simulink model "hak"  (R2023b)
settings: Solver=VariableStepAuto  StartTime=0.0  StopTime=10  RelTol=1e-3
libraries: mpclib x1, cstblocks x1
settings Model: Creator=serga  LastModifiedBy=serga

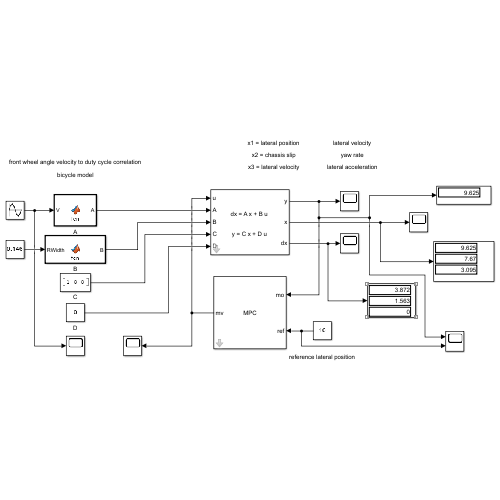
[thumbnail: Simulink's stored preview of the top-level diagram]
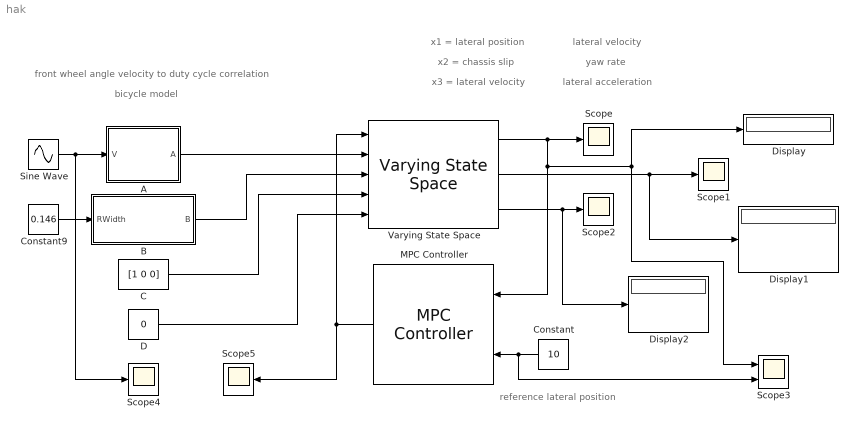
== system hak ==
  note: bicycle model
  note: front wheel angle velocity to duty cycle correlation
  note: reference lateral position
  note: lateral acceleration
  note: yaw rate
  note: lateral velocity
  note: x3 = lateral velocity
  note: x2 = chassis slip
  note: x1 = lateral position
  A : MATLAB Function  TreatAsAtomicUnit=on
  B : MATLAB Function  TreatAsAtomicUnit=on
  C : Constant  Value=[1 0 0]  VectorParams1D=off
  Constant : Constant  Value=10
  Constant9 : Constant  Value=0.146
  D : Constant  Value=0  VectorParams1D=off
  Display : Display
  Display1 : Display
  Display2 : Display
  MPC Controller : mpclib/MPC Controller  SCDEnableBlockLinearizationSpecification=on  mpcobj=mpc1  is_multiple=0  enable_value=0  return_u0=off  updateMPCinCallerWorkspace=on  md_inport=off  mv_inport=off  uref_inport=off  return_cost=off  return_mvseq=off  return_qpstatus=off  return_xseq=off  return_state=off  return_ovseq=off  state_inport=off  umin_inport=off  umax_inport=off  ymin_inport=off  ymax_inport=off  cc_inport=off  ywt_inport=off  uwt_inport=off  duwt_inport=off  rhoeps_inport=off  pm_inport=off  MaximumP=10  HorizonChoice=FixedHorizon  n_ts=0.1  n_p=50  n_mv=1  n_md=0  n_ud=0  n_mo=1  n_uo=0  BlockDataType=double  SampleTimeInherited=off  switch_inport=off
  Scope{,1..2,4..5} (5 alike) : Scope
  Scope3 : Scope  NumInputPorts=2
  Sine Wave : Sin  Amplitude=0.6  Frequency=0.1  SampleTime=0
  Varying State Space : cstblocks/Linear Parameter Varying/Varying State Space  x0=0  xNames=''  OutputX=on  OutputDX=on  Feedthrough=on
  wires:
  A/1(A) -> Varying State Space/2
  B/1(B) -> Varying State Space/3
  C/1 -> Varying State Space/4
  D/1 -> Varying State Space/5
  Constant9/1 -> B/1(RWidth)
  Varying State Space/1 -> MPC Controller/1, Display/1, Scope3/1, Scope/1
  Varying State Space/2 -> Display1/1, Scope1/1
  Varying State Space/3 -> Display2/1, Scope2/1
  MPC Controller/1 -> Scope5/1, Varying State Space/1
  Sine Wave/1 -> Scope4/1, A/1(V)
  Constant/1 -> Scope3/2, MPC Controller/2

== matlab function hak/B ==
  data: RWidth input; B output
function B = fcn(RWidth)

B = [0; ...
     0; ...
     1/RWidth];

== matlab function hak/A ==
  data: V input; A output
function A = fcn(V)

A = [0 V 0; ...
     0 0 V; ...
     0 0 0];
